simulink model "trocador_PS_GPC_GDMC_sim"  (R2020a)
settings: Solver=VariableStepAuto  StartTime=0.0  StopTime=tsim  MaxStep=0.01  RelTol=1e-3
values from neighbouring files (symbols this model uses):
  amppert = 0.5    [trocador_PS_GPC_GDMC.m]
  amppert2 = -0.1    [trocador_PS_GPC_GDMC.m]
  ampref = 1    [trocador_PS_GPC_GDMC.m]
  Fgpc = Ftemp    [trocador_PS_GPC_GDMC.m]
  Hgdmc = H1-H2    [trocador_PS_GPC_GDMC.m]    (also in trocador_PS_GPC_GDMC_bode.m; trocador_PS_GPC_GDMC_bode2.m)
  Hgpc = cell2mat(H)    [trocador_PS_GPC_GDMC.m]
  Kgdmc1 = Kgdmc(1,:)    [trocador_PS_GPC_GDMC.m]    (also in trocador_PS_GPC_GDMC_bode.m; trocador_PS_GPC_GDMC_bode2.m)
  Kgpc1 = [Kgpc1; Kgpc(sum(Nu(1:i-1))+1,:)]    [trocador_PS_GPC_GDMC.m]    (also in trocador_PS_GPC_GDMC_bode.m = Kgpc(1,:))
  tpert = 15    [trocador_PS_GPC_GDMC.m]
  tpert2 = 25    [trocador_PS_GPC_GDMC.m]
  tref = 4    [trocador_PS_GPC_GDMC.m]
  Ts = 0.15    [trocador_PS_GPC_GDMC.m]    (also in trocador_PS_GPC_GDMC_bode.m; trocador_PS_GPC_GDMC_bode2.m)
  zr = blkdiag(zr,ones(Ny(i),1))    [trocador_PS_GPC_GDMC.m]
libraries: cstblocks x11
settings Model: Creator=treezao  LastModifiedBy=treezao

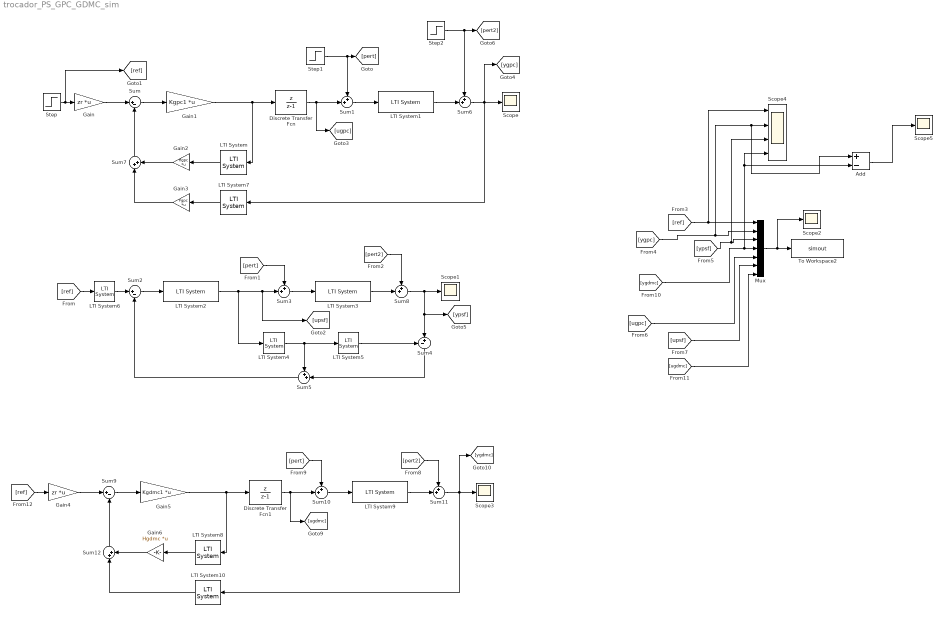
== system trocador_PS_GPC_GDMC_sim ==
  Add : Sum  Inputs=+-
  Discrete Transfer Fcn : DiscreteTransferFcn  Numerator=[1 0]  Denominator=[1 -1]  SampleTime=Ts
  Discrete Transfer Fcn1 : DiscreteTransferFcn  Numerator=[1 0]  Denominator=[1 -1]  SampleTime=Ts
  Gain : Gain  Gain=zr  Multiplication=Matrix(K*u)
  Gain1 : Gain  Gain=Kgpc1  Multiplication=Matrix(K*u)
  Gain2 : Gain  Gain=Hgpc  Multiplication=Matrix(K*u)
  Gain3 : Gain  Gain=Fgpc  Multiplication=Matrix(K*u)
  Gain4 : Gain  Gain=zr  Multiplication=Matrix(K*u)
  Gain5 : Gain  Gain=Kgdmc1  Multiplication=Matrix(K*u)
  Gain6 : Gain  Gain=Hgdmc  Multiplication=Matrix(K*u)
  LTI System : cstblocks/LTI System  sys=zu  IC=[]
  LTI System1 : cstblocks/LTI System  sys=P  IC=[]
  LTI System10 : cstblocks/LTI System  sys=Fegdmc  IC=[]
  LTI System2 : cstblocks/LTI System  sys=Czps  IC=[]
  LTI System3 : cstblocks/LTI System  sys=P  IC=[]
  LTI System4 : cstblocks/LTI System  sys=Gnz  IC=[]
  LTI System5 : cstblocks/LTI System  sys=Lnz  IC=[]
  LTI System6 : cstblocks/LTI System  sys=Fzps  IC=[]
  LTI System7 : cstblocks/LTI System  sys=zy  IC=[]
  LTI System8 : cstblocks/LTI System  sys=zudmc  IC=[]
  LTI System9 : cstblocks/LTI System  sys=P  IC=[]
  Mux : Mux  Inputs=7
  Scope{,1..3,5} (5 alike) : Scope
  Scope4 : Scope  NumInputPorts=4
  Step : Step  Time=tref  After=ampref  SampleTime=0
  Step1 : Step  Time=tpert  After=amppert  SampleTime=0
  Step2 : Step  Time=tpert2  After=amppert2  SampleTime=0
  Sum : Sum  Inputs=|+-
  Sum{1,3,5..6,8,10..11} (7 alike) : Sum  Inputs=++|
  Sum12 : Sum  Inputs=|++
  Sum2 : Sum  Inputs=|+-
  Sum4 : Sum  Inputs=-+|
  Sum7 : Sum  Inputs=|++
  Sum9 : Sum  Inputs=|+-
  To Workspace2 : ToWorkspace  VariableName=simout  SampleTime=-1
  wires:
  Step/1 -> [ref], Gain/1
  Sum/1 -> Gain1/1
  Gain1/1 -> LTI System/1, Discrete Transfer Fcn/1
  Step1/1 -> Sum1/1, [pert]
  Sum1/1 -> LTI System1/1
  Sum2/1 -> LTI System2/1
  [ref] -> LTI System6/1
  LTI System2/1 -> [upsf], Sum3/2, LTI System4/1
  Sum3/1 -> LTI System3/1
  [pert] -> Sum3/1
  LTI System4/1 -> Sum5/1, LTI System5/1
  LTI System5/1 -> Sum4/1
  Sum4/1 -> Sum5/2
  Sum5/1 -> Sum2/2
  Mux/1 -> Scope2/1, To Workspace2/1
  [ref] -> Scope4/1, Mux/1
  [ypsf] -> Scope4/3, Mux/3
  Step2/1 -> Sum6/1, [pert2]
  LTI System1/1 -> Sum6/2
  Sum6/1 -> LTI System7/1, [ygpc], Scope/1
  LTI System6/1 -> Sum2/1
  Gain/1 -> Sum/1
  Discrete Transfer Fcn/1 -> [ugpc], Sum1/2
  Sum7/1 -> Sum/2
  Gain2/1 -> Sum7/2
  LTI System/1 -> Gain2/1
  Gain3/1 -> Sum7/1
  LTI System7/1 -> Gain3/1
  LTI System3/1 -> Sum8/2
  Sum8/1 -> Sum4/2, [ypsf], Scope1/1
  [pert2] -> Sum8/1
  Sum11/1 -> LTI System10/1, [ygdmc], Scope3/1
  Gain6/1 -> Sum12/2
  LTI System8/1 -> Gain6/1
  Sum12/1 -> Sum9/2
  LTI System9/1 -> Sum11/2
  Gain5/1 -> LTI System8/1, Discrete Transfer Fcn1/1
  LTI System10/1 -> Sum12/1
  Gain4/1 -> Sum9/1
  Sum10/1 -> LTI System9/1
  Sum9/1 -> Gain5/1
  Discrete Transfer Fcn1/1 -> [ugdmc], Sum10/2
  [ref] -> Gain4/1
  [pert2] -> Sum11/1
  [pert] -> Sum10/1
  [ugpc] -> Mux/5
  [upsf] -> Mux/6
  [ygdmc] -> Add/2, Scope4/4, Mux/4
  [ugdmc] -> Mux/7
  [ygpc] -> Add/1, Scope4/2, Mux/2
  Add/1 -> Scope5/1
